simulink model "voltECMSBWD"  (R2022a)
settings: Solver=ode1  StartTime=0.0  StopTime=size(vrijeme,1)  FixedStep=1  EnableMultiTasking=on
values from neighbouring files (symbols this model uses):
  BLNDmode = 0    [main_Function.m]
  bufferSize = 28    [driving_cycle_load.m]
  chooseBound = 2    [main_Function.m]
  chooseControl = 0    [main_Function.m]
  chooseMode = 2    [main_Function.m]
  dekrement_SoC = 1*(0.3-0.95)/size(cpoints,1)    [driving_cycle_load.m]
  fix_hyst = 30    [main_Function.m]
  granicaPar = 48    [main_Function.m]
  hpg = 2.24    [initvolt.m]
  hystD = 30    [driving_cycle_load.m]
  hystG = 70    [driving_cycle_load.m]
  io = 2.16    [initvolt.m]
  Pbatt_charging = -10000    [main_Function.m]
  plugged_and_charging = 1    [main_Function.m]
  Qbat = 45*3600    (= 162000)    [initvolt.m]
  r = 0.3170    (= 0.317)    [initvolt.m]
  RBextended = 1    [main_Function.m]
  Rch = 0.056128    [initvolt.m]
  Rdch = 0.115904    [initvolt.m]
  Ssoc = 0.95    [initvolt.m]    (also in main_Function.m = 0.3)
  tcdstdD = 0    [driving_cycle_load.m]
  tcdstdG = 650    [driving_cycle_load.m]
undefined symbols (not defined in the file or in its folder): batsoc, mg1eff, mg2eff, Mmft, pgkor, pgsg, sgn, tuice, tuicemin, tumg1, tumg2
libraries: simulink x2
settings Model: Creator=novos  LastModifiedBy=novos
settings SolverCC: ZeroCrossControl=DisableAll
settings DataIOCC: LimitDataPoints=on  SaveFormat=Array  SignalLoggingSaveFormat=ModelDataLogs  ReturnWorkspaceOutputs=off  SignalLoggingName=sigsOut
settings OptimizationCC: InitFltsAndDblsToZero=on  LifeSpan=inf
settings DebuggingCC: SaveWithParameterizedLinksMsg=none  UnderspecifiedInitializationDetection=Classic  MergeDetectMultiDrivingBlocksExec=none  SignalResolutionControl=TryResolveAllWithWarning  MultiTaskDSMMsg=warning  MultiTaskCondExecSysMsg=none  UnconnectedInputMsg=warning  UnconnectedOutputMsg=warning  UnconnectedLineMsg=warning  SFUnexpectedBacktrackingDiag=warning  SFNoUnconditionalDefaultTransitionDiag=warning  SFExecutionAtInitializationDiag=none  SFMachineParentedDataDiag=warning  ArithmeticOperatorsInVariantConditions=warning
settings HardwareCC: ProdBitPerPointer=32  ProdBitPerSizeT=32  ProdBitPerPtrDiffT=32  ProdLargestAtomicFloat=None  ProdIntDivRoundTo=Undefined  ProdEndianess=Unspecified  ProdWordSize=32  ProdHWDeviceType=32-bit Generic  TargetUnknown=on
settings ModelReferenceCC: PropagateSignalLabelsOutOfModel=off
settings SFSimCC: SimUserSources=high_level_ctrl.c
settings CodeAppCC: StateflowObjectComments=on
settings GRTTargetCC: TargetFcnLib=ansi_tfl_tmw.mat  TargetLangStandard=C89/C90 (ANSI)  CombineOutputUpdateFcns=off  GRTInterface=on
settings ConfigComp: CovMetricSettings=dw  CovSaveCumulativeToWorkspaceVar=on  CovSaveSingleToWorkspaceVar=on

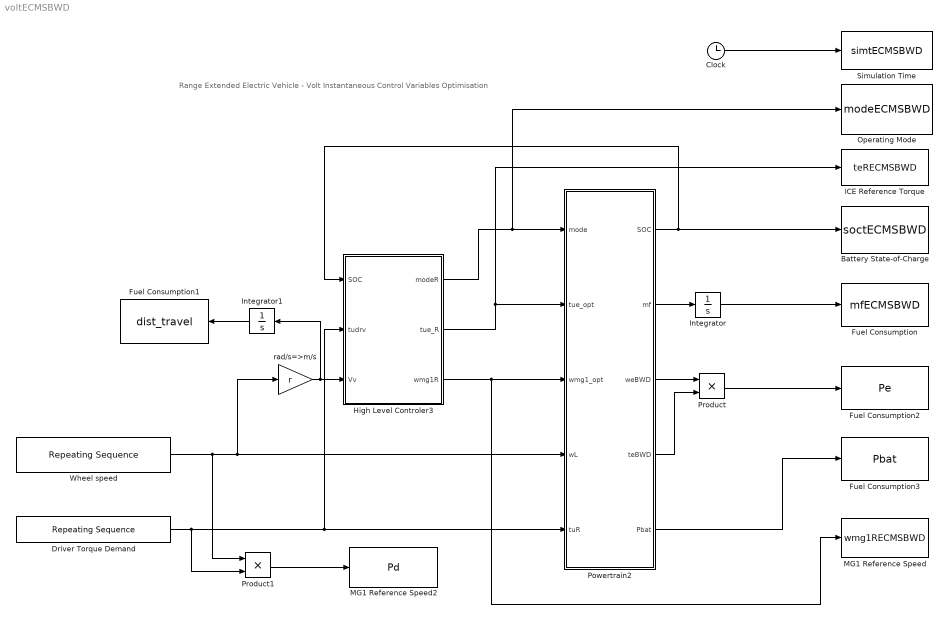
== system voltECMSBWD ==
  note: Range Extended Electric Vehicle - Volt Instantaneous Control Variables Optimisation
  Battery State-of-Charge : ToWorkspace  VariableName=soctECMSBWD  SampleTime=-1
  Clock : Clock
  Driver Torque Demand : simulink/Sources/Repeating Sequence  rep_seq_t=vrijeme  rep_seq_y=cmoment
  Fuel Consumption : ToWorkspace  VariableName=mfECMSBWD  SampleTime=-1
  Fuel Consumption1 : ToWorkspace  VariableName=dist_travel  SampleTime=-1
  Fuel Consumption2 : ToWorkspace  VariableName=Pe  SampleTime=-1
  Fuel Consumption3 : ToWorkspace  VariableName=Pbat  SampleTime=-1
  High Level Controler3 : Subsystem
  ICE Reference Torque : ToWorkspace  VariableName=teRECMSBWD  SampleTime=-1
  Integrator : Integrator
  Integrator1 : Integrator
  MG1 Reference Speed : ToWorkspace  VariableName=wmg1RECMSBWD  SampleTime=-1
  MG1 Reference Speed2 : ToWorkspace  VariableName=Pd  SampleTime=-1
  Operating Mode : ToWorkspace  VariableName=modeECMSBWD  SampleTime=-1
  Powertrain2 : Subsystem
  Product : Product  RndMeth=Zero
  Product1 : Product  RndMeth=Zero
  Simulation Time : ToWorkspace  VariableName=simtECMSBWD  SampleTime=-1
  Wheel speed : simulink/Sources/Repeating Sequence  rep_seq_t=vrijeme  rep_seq_y=cbrzina
  rad/s=>m/s : Gain  Gain=r  SaturateOnIntegerOverflow=on  OutDataTypeStr=Inherit: Same as input  ParamDataTypeStr=Inherit: Same as input
  wires:
  Powertrain2/1(SOC) -> Battery State-of-Charge/1, High Level Controler3/1(SOC)
  Powertrain2/2(mf) -> Integrator/1
  Clock/1 -> Simulation Time/1
  Wheel speed/1 -> Powertrain2/4(wL), rad/s=>m/s/1, Product1/1
  Driver Torque Demand/1 -> Powertrain2/5(tuR), High Level Controler3/2(tudrv), Product1/2
  Integrator/1 -> Fuel Consumption/1
  High Level Controler3/1(modeR) -> Powertrain2/1(mode), Operating Mode/1
  High Level Controler3/2(tue_R) -> Powertrain2/2(tue_opt), ICE Reference Torque/1
  High Level Controler3/3(wmg1R) -> Powertrain2/3(wmg1_opt), MG1 Reference Speed/1
  rad/s=>m/s/1 -> High Level Controler3/3(Vv), Integrator1/1
  Powertrain2/3(weBWD) -> Product/1
  Powertrain2/4(teBWD) -> Product/2
  Product/1 -> Fuel Consumption2/1
  Powertrain2/5(Pbat) -> Fuel Consumption3/1
  Product1/1 -> MG1 Reference Speed2/1
  Integrator1/1 -> Fuel Consumption1/1

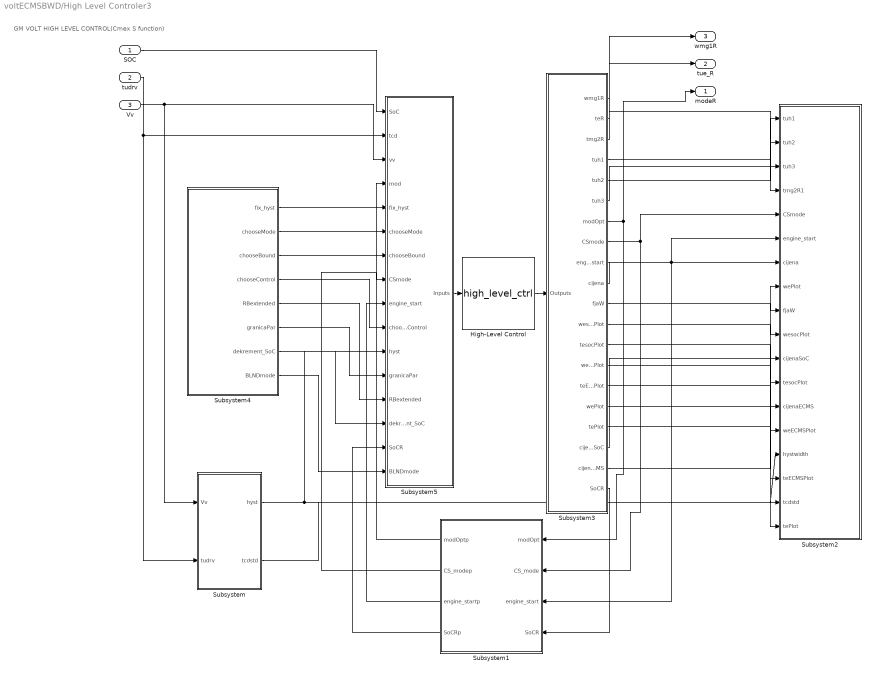
== system voltECMSBWD/High Level Controler3 ==
  note: GM VOLT HIGH LEVEL CONTROL(Cmex S function)
  SOC : Inport
  tudrv : Inport  Port=2
  Vv : Inport  Port=3
  High-Level Control : S-Function  FunctionName=high_level_ctrl  Parameters=Mmft, mg1eff, mg2eff  SFunctionDeploymentMode=off  EnableBusSupport=off
  Subsystem : Subsystem
  Subsystem1 : Subsystem
  Subsystem2 : Subsystem
  Subsystem3 : Subsystem
  Subsystem4 : Subsystem
  Subsystem5 : Subsystem
  modeR : Outport
  tue_R : Outport  Port=2
  wmg1R : Outport  Port=3
  wires:
  Subsystem3/7(modOpt) -> Subsystem1/1(modOpt), modeR/1
  Subsystem3/6(tuh3) -> Subsystem2/3(tuh3)
  Subsystem3/5(tuh2) -> Subsystem2/2(tuh2)
  Subsystem3/4(tuh1) -> Subsystem2/1(tuh1)
  Vv/1 -> Subsystem/1(Vv), Subsystem5/3(vv)
  tudrv/1 -> Subsystem/2(tudrv), Subsystem5/2(tcd)
  Subsystem3/3(tmg2R) -> Subsystem2/4(tmg2R1)
  Subsystem3/2(teR) -> tue_R/1
  Subsystem5/1(Inputs) -> High-Level Control/1
  High-Level Control/1 -> Subsystem3/1(Outputs)
  Subsystem3/9(engine_start) -> Subsystem1/3(engine_start), Subsystem2/6(engine_start)
  Subsystem3/8(CSmode) -> Subsystem1/2(CS_mode), Subsystem2/5(CSmode)
  Subsystem/1(hyst) -> Subsystem2/15(hystwidth), Subsystem5/11(hyst)
  Subsystem/2(tcdstd) -> Subsystem2/17(tcdstd)
  Subsystem3/10(cijena) -> Subsystem2/7(cijena)
  Subsystem3/11(fjaW) -> Subsystem2/9(fjaW)
  Subsystem3/12(wesocPlot) -> Subsystem2/10(wesocPlot)
  Subsystem3/13(tesocPlot) -> Subsystem2/12(tesocPlot)
  Subsystem3/14(weECMSPlot) -> Subsystem2/14(weECMSPlot)
  Subsystem3/15(teECMSPlot) -> Subsystem2/16(teECMSPlot)
  Subsystem3/17(tePlot) -> Subsystem2/18(tePlot)
  Subsystem3/18(cijenaSoC) -> Subsystem2/11(cijenaSoC)
  Subsystem3/19(cijenaECMS) -> Subsystem2/13(cijenaECMS)
  Subsystem3/1(wmg1R) -> wmg1R/1
  Subsystem3/20(SoCR) -> Subsystem1/4(SoCR)
  Subsystem3/16(wePlot) -> Subsystem2/8(wePlot)
  SOC/1 -> Subsystem5/1(SoC)
  Subsystem1/1(modOptp) -> Subsystem5/4(mod)
  Subsystem4/1(fix_hyst) -> Subsystem5/5(fix_hyst)
  Subsystem4/2(chooseMode) -> Subsystem5/6(chooseMode)
  Subsystem4/3(chooseBound) -> Subsystem5/7(chooseBound)
  Subsystem4/4(chooseControl) -> Subsystem5/10(chooseControl)
  Subsystem4/5(RBextended) -> Subsystem5/13(RBextended)
  Subsystem4/6(granicaPar) -> Subsystem5/12(granicaPar)
  Subsystem4/7(dekrement_SoC) -> Subsystem5/14(dekrement_SoC)
  Subsystem4/8(BLNDmode) -> Subsystem5/16(BLNDmode)
  Subsystem1/4(SoCRp) -> Subsystem5/15(SoCR)
  Subsystem1/3(engine_startp) -> Subsystem5/9(engine_start)
  Subsystem1/2(CS_modep) -> Subsystem5/8(CSmode)

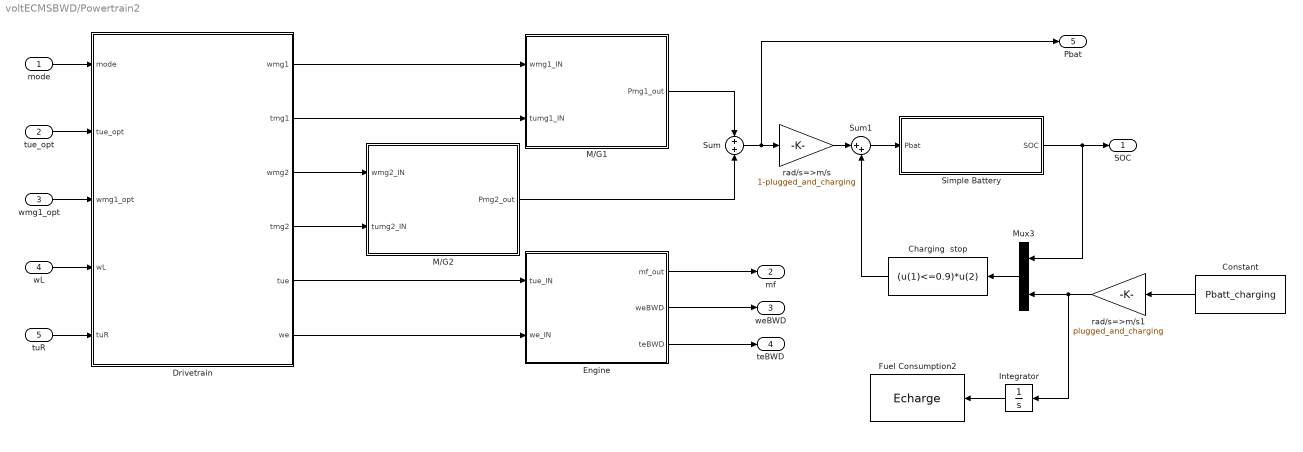
== system voltECMSBWD/Powertrain2 ==
  mode : Inport
  tue_opt : Inport  Port=2
  wmg1_opt : Inport  Port=3
  wL : Inport  Port=4
  tuR : Inport  Port=5
  Charging  stop : Fcn  Expr=(u(1)<=0.9)*u(2)
  Constant : Constant  Value=Pbatt_charging
  Drivetrain : Subsystem
  Engine : Subsystem
  Fuel Consumption2 : ToWorkspace  VariableName=Echarge  SampleTime=-1
  Integrator : Integrator
  M/G1 : Subsystem
  M/G2 : Subsystem
  Mux3 : Mux  Inputs=2
  Simple Battery : Subsystem
  Sum : Sum  SaturateOnIntegerOverflow=on
  Sum1 : Sum  Inputs=|++  SaturateOnIntegerOverflow=on
  rad/s=>m/s : Gain  Gain=1-plugged_and_charging  SaturateOnIntegerOverflow=on  OutDataTypeStr=Inherit: Same as input  ParamDataTypeStr=Inherit: Same as input
  rad/s=>m/s1 : Gain  Gain=plugged_and_charging  SaturateOnIntegerOverflow=on  OutDataTypeStr=Inherit: Same as input  ParamDataTypeStr=Inherit: Same as input
  SOC : Outport
  mf : Outport  Port=2
  weBWD : Outport  Port=3
  teBWD : Outport  Port=4
  Pbat : Outport  Port=5
  wires:
  Sum/1 -> Pbat/1, rad/s=>m/s/1
  M/G2/1(Pmg2_out) -> Sum/2
  Simple Battery/1(SOC) -> SOC/1, Mux3/1
  Engine/1(mf_out) -> mf/1
  M/G1/1(Pmg1_out) -> Sum/1
  mode/1 -> Drivetrain/1(mode)
  tue_opt/1 -> Drivetrain/2(tue_opt)
  wmg1_opt/1 -> Drivetrain/3(wmg1_opt)
  wL/1 -> Drivetrain/4(wL)
  tuR/1 -> Drivetrain/5(tuR)
  Drivetrain/1(wmg1) -> M/G1/1(wmg1_IN)
  Drivetrain/2(tmg1) -> M/G1/2(tumg1_IN)
  Drivetrain/3(wmg2) -> M/G2/1(wmg2_IN)
  Drivetrain/4(tmg2) -> M/G2/2(tumg2_IN)
  Drivetrain/5(tue) -> Engine/1(tue_IN)
  Drivetrain/6(we) -> Engine/2(we_IN)
  Engine/2(weBWD) -> weBWD/1
  Engine/3(teBWD) -> teBWD/1
  Sum1/1 -> Simple Battery/1(Pbat)
  Constant/1 -> rad/s=>m/s1/1
  Mux3/1 -> Charging  stop/1
  Charging  stop/1 -> Sum1/2
  rad/s=>m/s/1 -> Sum1/1
  rad/s=>m/s1/1 -> Mux3/2, Integrator/1
  Integrator/1 -> Fuel Consumption2/1

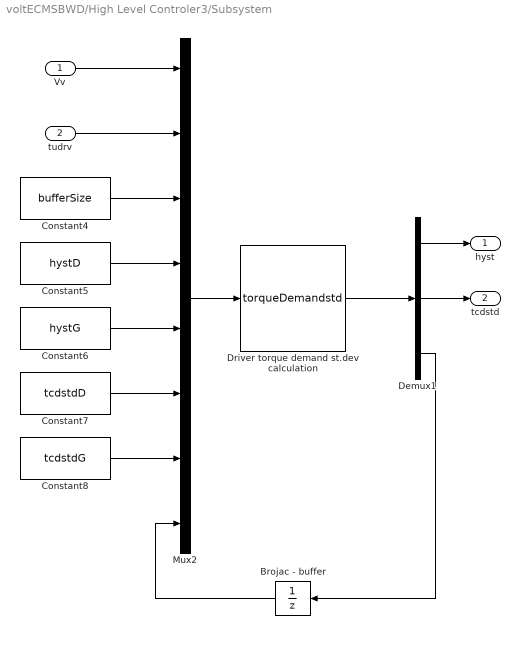
== system voltECMSBWD/High Level Controler3/Subsystem ==
  Vv : Inport
  tudrv : Inport  Port=2
  Brojac - buffer : UnitDelay  SampleTime=-1
  Constant4 : Constant  Value=bufferSize
  Constant5 : Constant  Value=hystD
  Constant6 : Constant  Value=hystG
  Constant7 : Constant  Value=tcdstdD
  Constant8 : Constant  Value=tcdstdG
  Demux1 : Demux  Outputs=3
  Driver torque demand st.dev calculation : S-Function  FunctionName=torqueDemandstd  SFunctionDeploymentMode=off  EnableBusSupport=off
  Mux2 : Mux  Inputs=8
  hyst : Outport
  tcdstd : Outport  Port=2
  wires:
  Mux2/1 -> Driver torque demand st.dev calculation/1
  Constant4/1 -> Mux2/3
  Driver torque demand st.dev calculation/1 -> Demux1/1
  Constant5/1 -> Mux2/4
  Constant6/1 -> Mux2/5
  Constant7/1 -> Mux2/6
  Constant8/1 -> Mux2/7
  Demux1/3 -> Brojac - buffer/1
  Vv/1 -> Mux2/1
  tudrv/1 -> Mux2/2
  Demux1/1 -> hyst/1
  Demux1/2 -> tcdstd/1
  Brojac - buffer/1 -> Mux2/8

== system voltECMSBWD/High Level Controler3/Subsystem1 ==
  modOpt : Inport
  CS_mode : Inport  Port=2
  engine_start : Inport  Port=3
  SoCR : Inport  Port=4
  Unit Delay : UnitDelay  SampleTime=-1
  Unit Delay 2 : UnitDelay  InitialCondition=Ssoc  SampleTime=-1
  Unit Delay 3 : UnitDelay  SampleTime=-1
  Unit Delay1 : UnitDelay  SampleTime=-1
  modOptp : Outport
  CS_modep : Outport  Port=2
  engine_startp : Outport  Port=3
  SoCRp : Outport  Port=4
  wires:
  modOpt/1 -> Unit Delay1/1
  CS_mode/1 -> Unit Delay/1
  engine_start/1 -> Unit Delay 3/1
  Unit Delay1/1 -> modOptp/1
  Unit Delay/1 -> CS_modep/1
  Unit Delay 3/1 -> engine_startp/1
  SoCR/1 -> Unit Delay 2/1
  Unit Delay 2/1 -> SoCRp/1

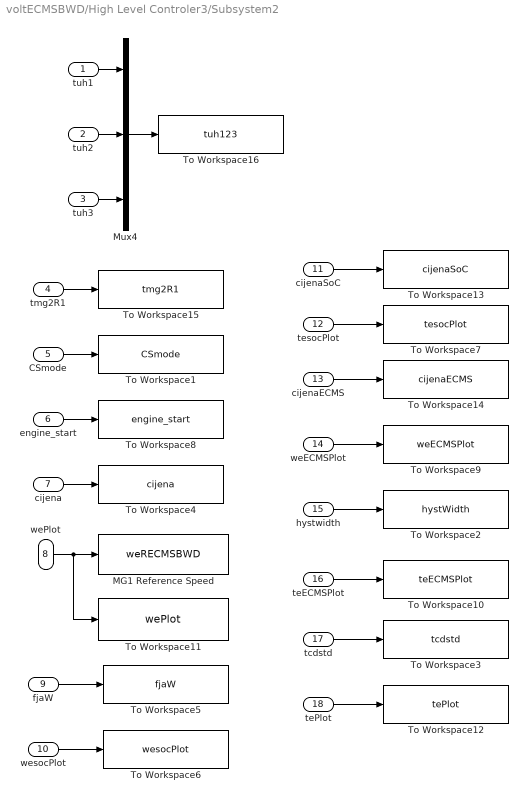
== system voltECMSBWD/High Level Controler3/Subsystem2 ==
  tuh1 : Inport
  tuh2 : Inport  Port=2
  tuh3 : Inport  Port=3
  tmg2R1 : Inport  Port=4
  CSmode : Inport  Port=5
  engine_start : Inport  Port=6
  cijena : Inport  Port=7
  wePlot : Inport  Port=8
  fjaW : Inport  Port=9
  wesocPlot : Inport  Port=10
  cijenaSoC : Inport  Port=11
  tesocPlot : Inport  Port=12
  cijenaECMS : Inport  Port=13
  weECMSPlot : Inport  Port=14
  hystwidth : Inport  Port=15
  teECMSPlot : Inport  Port=16
  tcdstd : Inport  Port=17
  tePlot : Inport  Port=18
  MG1 Reference Speed : ToWorkspace  VariableName=weRECMSBWD  SampleTime=-1
  Mux4 : Mux  Inputs=3
  To Workspace1 : ToWorkspace  VariableName=CSmode  SampleTime=-1
  To Workspace10 : ToWorkspace  VariableName=teECMSPlot
  To Workspace11 : ToWorkspace  VariableName=wePlot
  To Workspace12 : ToWorkspace  VariableName=tePlot
  To Workspace13 : ToWorkspace  VariableName=cijenaSoC
  To Workspace14 : ToWorkspace  VariableName=cijenaECMS
  To Workspace15 : ToWorkspace  VariableName=tmg2R1  SampleTime=-1
  To Workspace16 : ToWorkspace  VariableName=tuh123  SampleTime=-1
  To Workspace2 : ToWorkspace  VariableName=hystWidth  SampleTime=-1
  To Workspace3 : ToWorkspace  VariableName=tcdstd  SampleTime=-1
  To Workspace4 : ToWorkspace  VariableName=cijena
  To Workspace5 : ToWorkspace  VariableName=fjaW
  To Workspace6 : ToWorkspace  VariableName=wesocPlot
  To Workspace7 : ToWorkspace  VariableName=tesocPlot
  To Workspace8 : ToWorkspace  VariableName=engine_start  SampleTime=-1
  To Workspace9 : ToWorkspace  VariableName=weECMSPlot
  wires:
  Mux4/1 -> To Workspace16/1
  wePlot/1 -> MG1 Reference Speed/1, To Workspace11/1
  CSmode/1 -> To Workspace1/1
  engine_start/1 -> To Workspace8/1
  hystwidth/1 -> To Workspace2/1
  tuh1/1 -> Mux4/1
  tuh2/1 -> Mux4/2
  tuh3/1 -> Mux4/3
  tmg2R1/1 -> To Workspace15/1
  cijena/1 -> To Workspace4/1
  fjaW/1 -> To Workspace5/1
  wesocPlot/1 -> To Workspace6/1
  cijenaSoC/1 -> To Workspace13/1
  tesocPlot/1 -> To Workspace7/1
  cijenaECMS/1 -> To Workspace14/1
  weECMSPlot/1 -> To Workspace9/1
  teECMSPlot/1 -> To Workspace10/1
  tcdstd/1 -> To Workspace3/1
  tePlot/1 -> To Workspace12/1

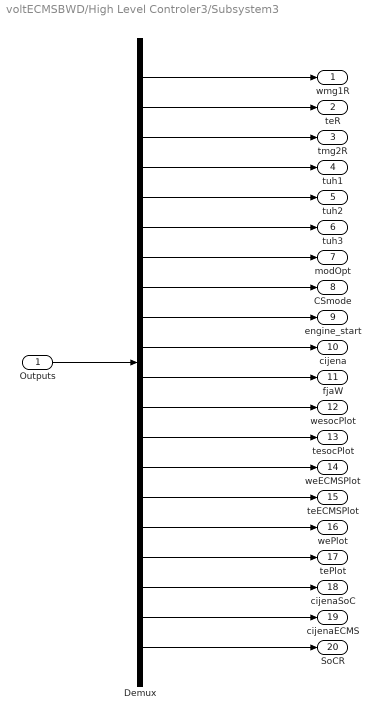
== system voltECMSBWD/High Level Controler3/Subsystem3 ==
  Outputs : Inport
  Demux : Demux  Outputs=20
  wmg1R : Outport
  teR : Outport  Port=2
  tmg2R : Outport  Port=3
  tuh1 : Outport  Port=4
  tuh2 : Outport  Port=5
  tuh3 : Outport  Port=6
  modOpt : Outport  Port=7
  CSmode : Outport  Port=8
  engine_start : Outport  Port=9
  cijena : Outport  Port=10
  fjaW : Outport  Port=11
  wesocPlot : Outport  Port=12
  tesocPlot : Outport  Port=13
  weECMSPlot : Outport  Port=14
  teECMSPlot : Outport  Port=15
  wePlot : Outport  Port=16
  tePlot : Outport  Port=17
  cijenaSoC : Outport  Port=18
  cijenaECMS : Outport  Port=19
  SoCR : Outport  Port=20
  wires:
  Demux/1 -> wmg1R/1
  Demux/2 -> teR/1
  Demux/3 -> tmg2R/1
  Demux/4 -> tuh1/1
  Demux/5 -> tuh2/1
  Demux/6 -> tuh3/1
  Demux/7 -> modOpt/1
  Demux/8 -> CSmode/1
  Demux/9 -> engine_start/1
  Demux/10 -> cijena/1
  Outputs/1 -> Demux/1
  Demux/11 -> fjaW/1
  Demux/12 -> wesocPlot/1
  Demux/13 -> tesocPlot/1
  Demux/14 -> weECMSPlot/1
  Demux/15 -> teECMSPlot/1
  Demux/16 -> wePlot/1
  Demux/17 -> tePlot/1
  Demux/18 -> cijenaSoC/1
  Demux/19 -> cijenaECMS/1
  Demux/20 -> SoCR/1

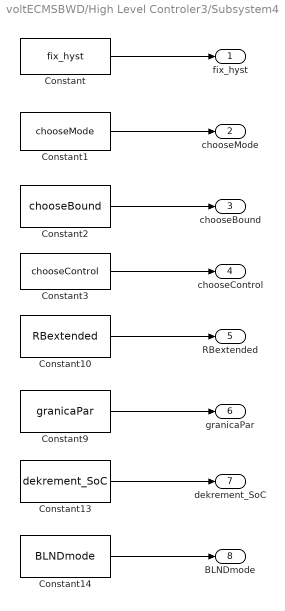
== system voltECMSBWD/High Level Controler3/Subsystem4 ==
  Constant : Constant  Value=fix_hyst
  Constant1 : Constant  Value=chooseMode
  Constant10 : Constant  Value=RBextended
  Constant13 : Constant  Value=dekrement_SoC
  Constant14 : Constant  Value=BLNDmode
  Constant2 : Constant  Value=chooseBound
  Constant3 : Constant  Value=chooseControl
  Constant9 : Constant  Value=granicaPar
  fix_hyst : Outport
  chooseMode : Outport  Port=2
  chooseBound : Outport  Port=3
  chooseControl : Outport  Port=4
  RBextended : Outport  Port=5
  granicaPar : Outport  Port=6
  dekrement_SoC : Outport  Port=7
  BLNDmode : Outport  Port=8
  wires:
  Constant/1 -> fix_hyst/1
  Constant1/1 -> chooseMode/1
  Constant2/1 -> chooseBound/1
  Constant3/1 -> chooseControl/1
  Constant10/1 -> RBextended/1
  Constant9/1 -> granicaPar/1
  Constant13/1 -> dekrement_SoC/1
  Constant14/1 -> BLNDmode/1

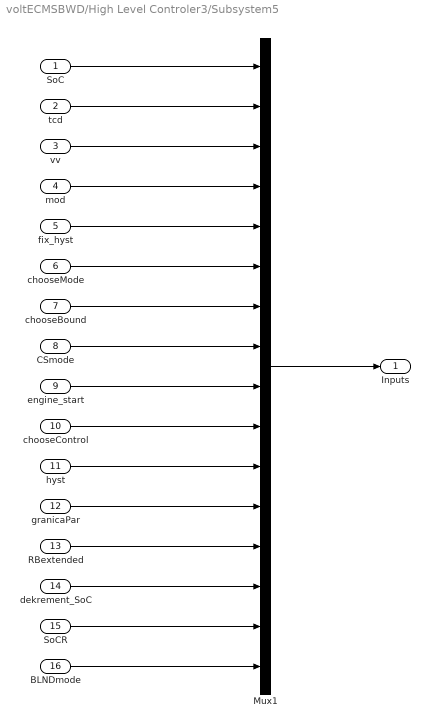
== system voltECMSBWD/High Level Controler3/Subsystem5 ==
  SoC : Inport
  tcd : Inport  Port=2
  vv : Inport  Port=3
  mod : Inport  Port=4
  fix_hyst : Inport  Port=5
  chooseMode : Inport  Port=6
  chooseBound : Inport  Port=7
  CSmode : Inport  Port=8
  engine_start : Inport  Port=9
  chooseControl : Inport  Port=10
  hyst : Inport  Port=11
  granicaPar : Inport  Port=12
  RBextended : Inport  Port=13
  dekrement_SoC : Inport  Port=14
  SoCR : Inport  Port=15
  BLNDmode : Inport  Port=16
  Mux1 : Mux  Inputs=16
  Inputs : Outport
  wires:
  tcd/1 -> Mux1/2
  vv/1 -> Mux1/3
  hyst/1 -> Mux1/11
  SoC/1 -> Mux1/1
  mod/1 -> Mux1/4
  fix_hyst/1 -> Mux1/5
  chooseMode/1 -> Mux1/6
  chooseBound/1 -> Mux1/7
  CSmode/1 -> Mux1/8
  Mux1/1 -> Inputs/1
  engine_start/1 -> Mux1/9
  chooseControl/1 -> Mux1/10
  granicaPar/1 -> Mux1/12
  RBextended/1 -> Mux1/13
  dekrement_SoC/1 -> Mux1/14
  SoCR/1 -> Mux1/15
  BLNDmode/1 -> Mux1/16

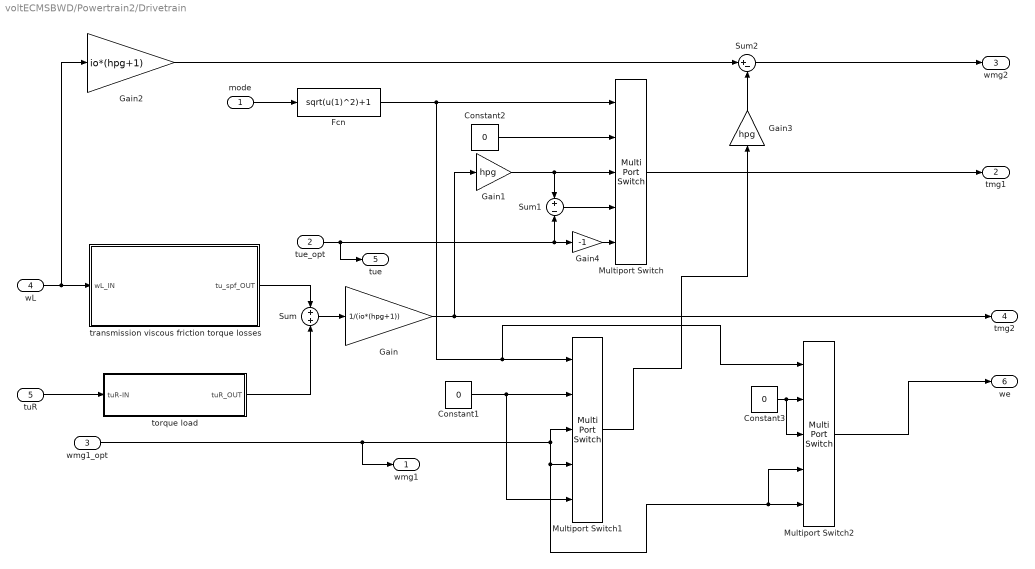
== system voltECMSBWD/Powertrain2/Drivetrain ==
  mode : Inport
  tue_opt : Inport  Port=2
  wmg1_opt : Inport  Port=3
  wL : Inport  Port=4
  tuR : Inport  Port=5
  Constant1 : Constant  Value=0
  Constant2 : Constant  Value=0
  Constant3 : Constant  Value=0
  Fcn : Fcn  Expr=sqrt(u(1)^2)+1
  Gain : Gain  Gain=1/(io*(hpg+1))
  Gain1 : Gain  Gain=hpg
  Gain2 : Gain  Gain=io*(hpg+1)
  Gain3 : Gain  Gain=hpg
  Gain4 : Gain  Gain=-1
  Multiport Switch : MultiPortSwitch  Inputs=4  InputSameDT=off
  Multiport Switch1 : MultiPortSwitch  Inputs=4  InputSameDT=off
  Multiport Switch2 : MultiPortSwitch  Inputs=4  InputSameDT=off
  Sum : Sum  SaturateOnIntegerOverflow=on
  Sum1 : Sum  Inputs=+-  SaturateOnIntegerOverflow=on
  Sum2 : Sum  Inputs=|+-  SaturateOnIntegerOverflow=on
  torque load : Subsystem
  transmission viscous friction torque losses : Subsystem
  wmg1 : Outport
  tmg1 : Outport  Port=2
  wmg2 : Outport  Port=3
  tmg2 : Outport  Port=4
  tue : Outport  Port=5
  we : Outport  Port=6
  wires:
  tuR/1 -> torque load/1(tuR-IN)
  transmission viscous friction torque losses/1(tu_spf_OUT) -> Sum/1
  wL/1 -> transmission viscous friction torque losses/1(wL_IN), Gain2/1
  mode/1 -> Fcn/1
  Sum/1 -> Gain/1
  Gain/1 -> Gain1/1, tmg2/1
  Fcn/1 -> Multiport Switch/1, Multiport Switch1/1, Multiport Switch2/1
  wmg1_opt/1 -> Multiport Switch1/3, Multiport Switch1/4, Multiport Switch2/5, Multiport Switch2/4, wmg1/1
  Gain1/1 -> Multiport Switch/3, Sum1/1
  Constant2/1 -> Multiport Switch/2
  tue_opt/1 -> Sum1/2, Gain4/1, tue/1
  Multiport Switch/1 -> tmg1/1
  Sum1/1 -> Multiport Switch/4
  Constant1/1 -> Multiport Switch1/2, Multiport Switch1/5
  Multiport Switch1/1 -> Gain3/1
  Constant3/1 -> Multiport Switch2/2, Multiport Switch2/3
  Multiport Switch2/1 -> we/1
  Gain2/1 -> Sum2/1
  Sum2/1 -> wmg2/1
  Gain3/1 -> Sum2/2
  Gain4/1 -> Multiport Switch/5
  torque load/1(tuR_OUT) -> Sum/2

== system voltECMSBWD/Powertrain2/Engine ==
  tue_IN : Inport
  we_IN : Inport  Port=2
  Fuel Consumption : ToWorkspace  VariableName=Pe_stat  SampleTime=-1
  Fuel Consumption1 : ToWorkspace  VariableName=mf_stat  SampleTime=-1
  Mux : Mux  Inputs=3
  Product : Product  RndMeth=Zero
  mf_map : Lookup2D  DialogController=Simulink.DDGSource  RowIndex=[1:size(Mmft,1)]  ColumnIndex=[1:size(Mmft,2)]  Table=Mmft  InputSameDT=off
  tue_MAX : Lookup  DialogController=Simulink.DDGSource  InputValues=tuice(:,1)  Table=tuice(:,2)
  tue_MIN : Lookup  DialogController=Simulink.DDGSource  InputValues=tuicemin(:,1)  Table=tuicemin(:,2)
  tue_MIN<tue<tue_MAX : Fcn  Expr=u(1)*(u(1)<u(2))*(u(1)>u(3))+u(2)*(u(1)>=u(2))+u(3)*(u(1)<=u(3))
  mf_out : Outport
  weBWD : Outport  Port=2
  teBWD : Outport  Port=3
  wires:
  we_IN/1 -> tue_MIN/1, tue_MAX/1, mf_map/2, weBWD/1, Product/1
  mf_map/1 -> mf_out/1, Fuel Consumption1/1
  tue_MIN/1 -> Mux/3
  tue_MAX/1 -> Mux/2
  tue_IN/1 -> Mux/1
  tue_MIN<tue<tue_MAX/1 -> mf_map/1, teBWD/1, Product/2
  Mux/1 -> tue_MIN<tue<tue_MAX/1
  Product/1 -> Fuel Consumption/1

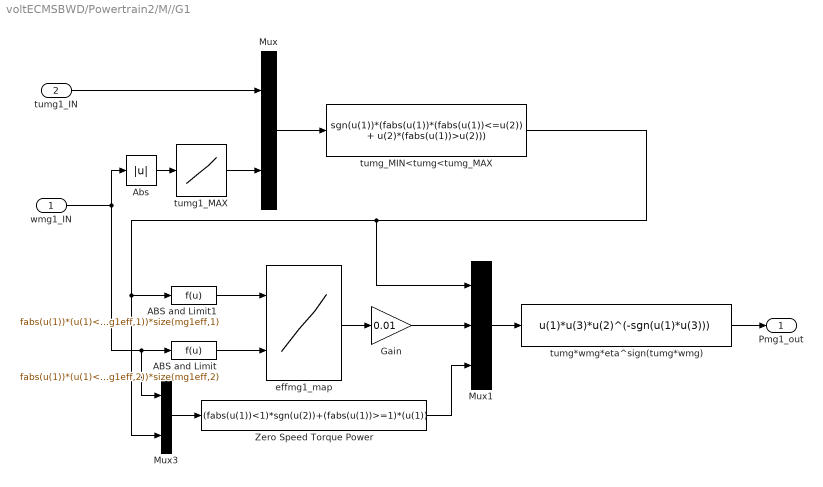
== system voltECMSBWD/Powertrain2/M//G1 ==
  wmg1_IN : Inport
  tumg1_IN : Inport  Port=2
  ABS and Limit : Fcn  Expr=fabs(u(1))*(u(1)<=size(mg1eff,2))+(u(1)>size(mg1eff,2))*size(mg1eff,2)
  ABS and Limit1 : Fcn  Expr=fabs(u(1))*(u(1)<=size(mg1eff,1))+(u(1)>size(mg1eff,1))*size(mg1eff,1)
  Abs : Abs
  Gain : Gain  Gain=0.01  SaturateOnIntegerOverflow=on  OutDataTypeStr=Inherit: Same as input  ParamDataTypeStr=Inherit: Same as input
  Mux : Mux  Inputs=2
  Mux1 : Mux  Inputs=3
  Mux3 : Mux  Inputs=2
  Zero Speed Torque Power : Fcn  Expr=(fabs(u(1))<1)*sgn(u(2))+(fabs(u(1))>=1)*(u(1))
  effmg1_map : Lookup2D  DialogController=Simulink.DDGSource  RowIndex=[0:size(mg1eff,1)-1]  ColumnIndex=[0:size(mg1eff,2)-1]  Table=mg1eff  InputSameDT=off
  tumg*wmg*eta^sign(tumg*wmg) : Fcn  Expr=u(1)*u(3)*u(2)^(-sgn(u(1)*u(3)))
  tumg1_MAX : Lookup  DialogController=Simulink.DDGSource  InputValues=[tumg1(:,1)' 2000]  Table=[tumg1(:,2)' 0]
  tumg_MIN<tumg<tumg_MAX : Fcn  Expr=sgn(u(1))*(fabs(u(1))*(fabs(u(1))<=u(2)) + u(2)*(fabs(u(1))>u(2)))
  Pmg1_out : Outport
  wires:
  wmg1_IN/1 -> Abs/1, ABS and Limit/1, Mux3/1
  effmg1_map/1 -> Gain/1
  tumg1_IN/1 -> Mux/1
  ABS and Limit/1 -> effmg1_map/2
  Gain/1 -> Mux1/2
  Mux1/1 -> tumg*wmg*eta^sign(tumg*wmg)/1
  tumg*wmg*eta^sign(tumg*wmg)/1 -> Pmg1_out/1
  ABS and Limit1/1 -> effmg1_map/1
  Zero Speed Torque Power/1 -> Mux1/3
  Mux3/1 -> Zero Speed Torque Power/1
  tumg_MIN<tumg<tumg_MAX/1 -> Mux1/1, ABS and Limit1/1, Mux3/2
  Abs/1 -> tumg1_MAX/1
  tumg1_MAX/1 -> Mux/2
  Mux/1 -> tumg_MIN<tumg<tumg_MAX/1

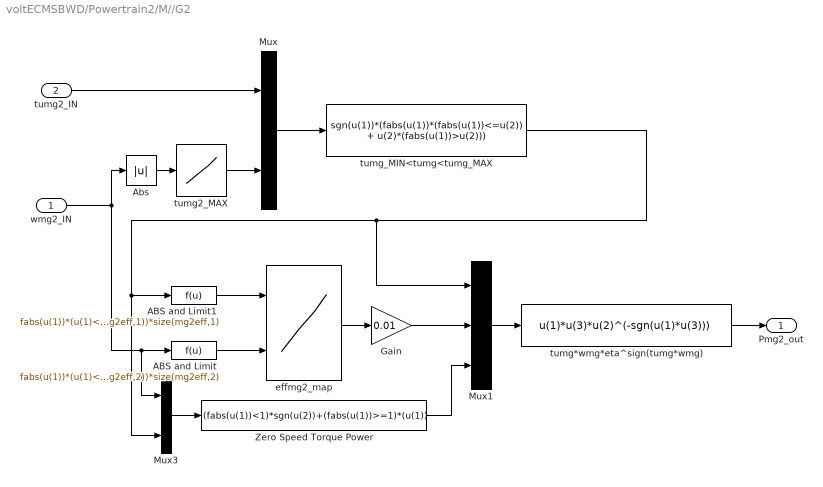
== system voltECMSBWD/Powertrain2/M//G2 ==
  wmg2_IN : Inport
  tumg2_IN : Inport  Port=2
  ABS and Limit : Fcn  Expr=fabs(u(1))*(u(1)<=size(mg2eff,2))+(u(1)>size(mg2eff,2))*size(mg2eff,2)
  ABS and Limit1 : Fcn  Expr=fabs(u(1))*(u(1)<=size(mg2eff,1))+(u(1)>size(mg2eff,1))*size(mg2eff,1)
  Abs : Abs
  Gain : Gain  Gain=0.01  SaturateOnIntegerOverflow=on  OutDataTypeStr=Inherit: Same as input  ParamDataTypeStr=Inherit: Same as input
  Mux : Mux  Inputs=2
  Mux1 : Mux  Inputs=3
  Mux3 : Mux  Inputs=2
  Zero Speed Torque Power : Fcn  Expr=(fabs(u(1))<1)*sgn(u(2))+(fabs(u(1))>=1)*(u(1))
  effmg2_map : Lookup2D  DialogController=Simulink.DDGSource  RowIndex=[0:size(mg2eff,1)-1]  ColumnIndex=[0:size(mg2eff,2)-1]  Table=mg2eff  InputSameDT=off
  tumg*wmg*eta^sign(tumg*wmg) : Fcn  Expr=u(1)*u(3)*u(2)^(-sgn(u(1)*u(3)))
  tumg2_MAX : Lookup  DialogController=Simulink.DDGSource  InputValues=[tumg2(:,1)' 2000]  Table=[tumg2(:,2)' 0]
  tumg_MIN<tumg<tumg_MAX : Fcn  Expr=sgn(u(1))*(fabs(u(1))*(fabs(u(1))<=u(2)) + u(2)*(fabs(u(1))>u(2)))
  Pmg2_out : Outport
  wires:
  wmg2_IN/1 -> Abs/1, ABS and Limit/1, Mux3/1
  effmg2_map/1 -> Gain/1
  tumg2_IN/1 -> Mux/1
  ABS and Limit/1 -> effmg2_map/2
  Gain/1 -> Mux1/2
  Mux1/1 -> tumg*wmg*eta^sign(tumg*wmg)/1
  tumg*wmg*eta^sign(tumg*wmg)/1 -> Pmg2_out/1
  ABS and Limit1/1 -> effmg2_map/1
  Zero Speed Torque Power/1 -> Mux1/3
  Mux3/1 -> Zero Speed Torque Power/1
  tumg_MIN<tumg<tumg_MAX/1 -> Mux1/1, ABS and Limit1/1, Mux3/2
  Mux/1 -> tumg_MIN<tumg<tumg_MAX/1
  tumg2_MAX/1 -> Mux/2
  Abs/1 -> tumg2_MAX/1

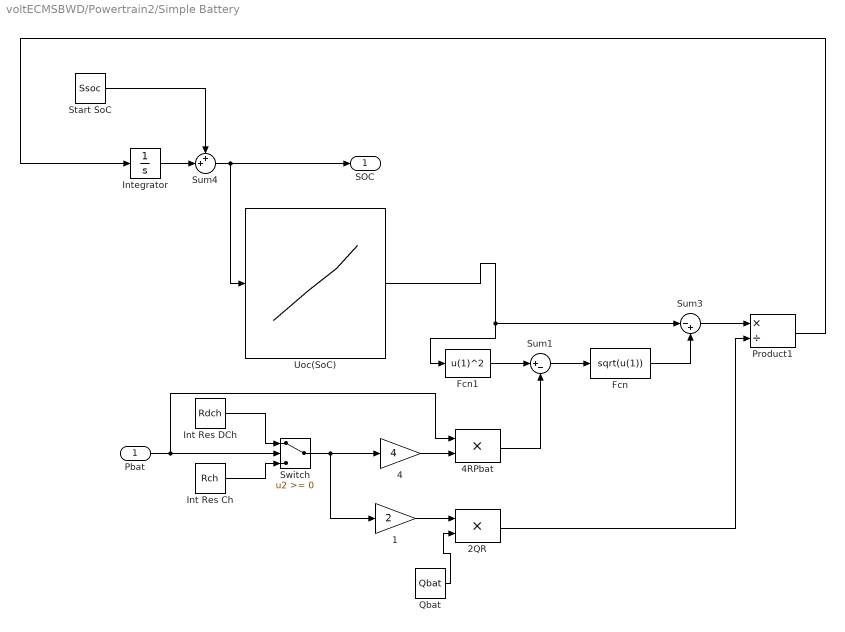
== system voltECMSBWD/Powertrain2/Simple Battery ==
  Pbat : Inport
  1 : Gain  Gain=2  SaturateOnIntegerOverflow=on  OutDataTypeStr=Inherit: Same as input  ParamDataTypeStr=Inherit: Same as input
  2QR : Product  SaturateOnIntegerOverflow=on  OutDataTypeStr=Inherit: Same as first input
  4 : Gain  Gain=4  SaturateOnIntegerOverflow=on  OutDataTypeStr=Inherit: Same as input  ParamDataTypeStr=Inherit: Same as input
  4RPbat : Product  SaturateOnIntegerOverflow=on  OutDataTypeStr=Inherit: Same as first input
  Fcn : Fcn  Expr=sqrt(u(1))
  Fcn1 : Fcn  Expr=u(1)^2
  Int Res Ch : Constant  Value=Rch
  Int Res DCh : Constant  Value=Rdch
  Integrator : Integrator
  Product1 : Product  Inputs=*/  SaturateOnIntegerOverflow=on  OutDataTypeStr=Inherit: Same as first input
  Qbat : Constant  Value=Qbat
  Start SoC : Constant  Value=Ssoc
  Sum1 : Sum  Inputs=|+-  SaturateOnIntegerOverflow=on
  Sum3 : Sum  Inputs=|-+  SaturateOnIntegerOverflow=on
  Sum4 : Sum  Inputs=++|  SaturateOnIntegerOverflow=on
  Switch : Switch  InputSameDT=off
  Uoc(SoC) : Lookup  DialogController=Simulink.DDGSource  InputValues=batsoc(:,1)  Table=batsoc(:,2)  LookUpMeth=Interpolation-Use End Values
  SOC : Outport
  wires:
  Pbat/1 -> Switch/2, 4RPbat/1
  Integrator/1 -> Sum4/2
  Start SoC/1 -> Sum4/1
  Sum4/1 -> SOC/1, Uoc(SoC)/1
  Fcn/1 -> Sum3/2
  Fcn1/1 -> Sum1/1
  Sum1/1 -> Fcn/1
  4RPbat/1 -> Sum1/2
  Sum3/1 -> Product1/1
  Product1/1 -> Integrator/1
  2QR/1 -> Product1/2
  Int Res Ch/1 -> Switch/3
  Int Res DCh/1 -> Switch/1
  Switch/1 -> 4/1, 1/1
  4/1 -> 4RPbat/2
  1/1 -> 2QR/1
  Qbat/1 -> 2QR/2
  Uoc(SoC)/1 -> Fcn1/1, Sum3/1

== system voltECMSBWD/Powertrain2/Drivetrain/torque load ==
  tuR-IN : Inport
  Abs1 : Abs
  Product3 : Product  Inputs=*/  SaturateOnIntegerOverflow=on  OutDataTypeStr=Inherit: Same as first input
  pg1 : Lookup  DialogController=Simulink.DDGSource  InputValues=pgkor(:,1)  Table=pgkor(:,2)  LookUpMeth=Interpolation-Use End Values
  tuR_OUT : Outport
  wires:
  Abs1/1 -> pg1/1
  pg1/1 -> Product3/2
  tuR-IN/1 -> Abs1/1, Product3/1
  Product3/1 -> tuR_OUT/1

== system voltECMSBWD/Powertrain2/Drivetrain/transmission viscous friction torque losses ==
  wL_IN : Inport
  Abs : Abs
  "Avoid \"Divide By Zero\"" : Fcn  Expr=(u(1)<0.1)*0.1+(u(1)>=0.1)*u(1)
  Pgub1 : Lookup  DialogController=Simulink.DDGSource  InputValues=pgsg(:,1)  Table=pgsg(:,2)
  Product4 : Product  Inputs=*/*  SaturateOnIntegerOverflow=on  OutDataTypeStr=Inherit: Same as first input
  Sign : Signum
  tu_spf_OUT : Outport
  wires:
  wL_IN/1 -> Sign/1, Abs/1
  Abs/1 -> Pgub1/1, "Avoid \"Divide By Zero\""/1
  Pgub1/1 -> Product4/1
  "Avoid \"Divide By Zero\""/1 -> Product4/2
  Sign/1 -> Product4/3
  Product4/1 -> tu_spf_OUT/1
